simulink model "Human_Intetion"  (R2020a)
settings: Solver=VariableStepAuto  StartTime=0.0  StopTime=10.0  RelTol=1e-3
values from neighbouring files (symbols this model uses):
  Fc_h = 5    [Teleop_parameters.m]    (also in base.mat; base_no_attrito.mat; ci_siamo.mat; force_control.mat)
  Kd_h = 0.5    [Teleop_parameters.m]    (also in base.mat = 1; base_no_attrito.mat = 1; ci_siamo.mat = 10; force_control.mat = 1)
  Kp_h = 1.2    [Teleop_parameters.m]    (also in base.mat; base_no_attrito.mat; ci_siamo.mat = 10; force_control.mat)
settings Model: Creator=gbagolin  LastModifiedBy=gbagolin

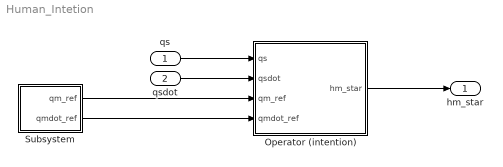
== system Human_Intetion ==
  qs : Inport
  qsdot : Inport  Port=2
  Operator (intention) : Subsystem
  Subsystem : Subsystem
  hm_star : Outport
  wires:
  qsdot/1 -> Operator (intention)/2(qsdot)
  Subsystem/2(qmdot_ref) -> Operator (intention)/4(qmdot_ref)
  Operator (intention)/1(hm_star) -> hm_star/1
  Subsystem/1(qm_ref) -> Operator (intention)/3(qm_ref)
  qs/1 -> Operator (intention)/1(qs)

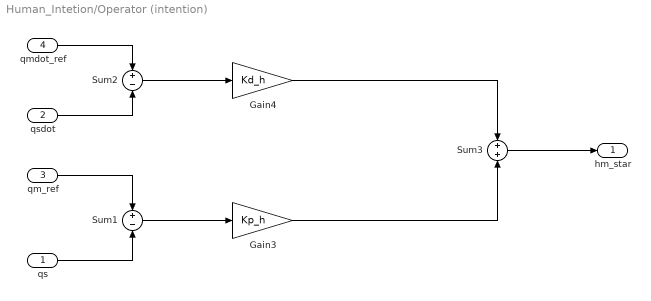
== system Human_Intetion/Operator (intention) ==
  qs : Inport
  qsdot : Inport  Port=2
  qm_ref : Inport  Port=3
  qmdot_ref : Inport  Port=4
  Gain3 : Gain  Gain=Kp_h
  Gain4 : Gain  Gain=Kd_h
  Sum1 : Sum  Inputs=+|-
  Sum2 : Sum  Inputs=+|-
  Sum3 : Sum  Inputs=+|+
  hm_star : Outport  VectorParamsAs1DForOutWhenUnconnected=off
  wires:
  qs/1 -> Sum1/2
  qm_ref/1 -> Sum1/1
  qmdot_ref/1 -> Sum2/1
  Sum1/1 -> Gain3/1
  qsdot/1 -> Sum2/2
  Sum2/1 -> Gain4/1
  Gain4/1 -> Sum3/1
  Gain3/1 -> Sum3/2
  Sum3/1 -> hm_star/1

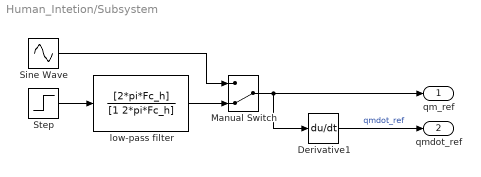
== system Human_Intetion/Subsystem ==
  Derivative1 : Derivative  CoefficientInTFapproximation=0.001
  Manual Switch : ManualSwitch  CurrentSetting=0
  Sine Wave : Sin  SampleTime=0
  Step : Step  SampleTime=0
  low-pass filter : TransferFcn  Numerator=[2*pi*Fc_h]  Denominator=[1 2*pi*Fc_h]
  qm_ref : Outport
  qmdot_ref : Outport  Port=2
  wires:
  low-pass filter/1 -> Manual Switch/2
  Manual Switch/1 -> qm_ref/1, Derivative1/1
  Derivative1/1 -> qmdot_ref/1  "qmdot_ref"
  Step/1 -> low-pass filter/1
  Sine Wave/1 -> Manual Switch/1
